simulink model "ECONANAL"  (Simulink 4.00)
settings: Solver=VariableStepDiscrete  SolverMode=SingleTasking  StartTime=0.0  StopTime=0  FixedStep=0  MaxStep=1  RelTol=1e-3  AbsTol=1e-6
settings Model: SaveTime=off  SaveOutput=off  LimitDataPoints=off  RTWTemplateMakefile=grt_unix.tmf  BlockReductionOpt=off

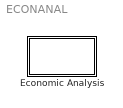
== system ECONANAL ==
  Economic Analysis : Subsystem
      settings: RTWFcnNameOpts=Auto  RTWFileNameOpts=Auto

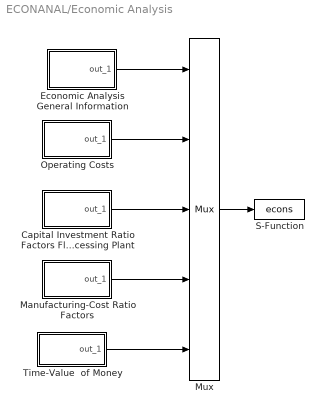
== system ECONANAL/Economic Analysis ==
  Capital Investment Ratio Factors Fluid Processing Plant : Subsystem
      settings: RTWFcnNameOpts=Auto  RTWFileNameOpts=Auto
  Economic Analysis General Information : Subsystem
      settings: RTWFcnNameOpts=Auto  RTWFileNameOpts=Auto
  Manufacturing-Cost Ratio Factors : Subsystem
      settings: RTWFcnNameOpts=Auto  RTWFileNameOpts=Auto
  Mux : Mux  Inputs=5
      settings: DisplayOption=none
  Operating Costs : Subsystem
      settings: RTWFcnNameOpts=Auto  RTWFileNameOpts=Auto
  S-Function : S-Function  FunctionName=econs  Parameters='ojstreams' 'ojunits'  PortCounts=[]  SFunctionModules=''
  Time-Value  of Money : Subsystem
      settings: RTWFcnNameOpts=Auto  RTWFileNameOpts=Auto
  wires:
  Economic Analysis General Information/1(out_1) -> Mux/1
  Mux/1 -> S-Function/1
  Time-Value  of Money/1(out_1) -> Mux/5
  Manufacturing-Cost Ratio Factors/1(out_1) -> Mux/4
  Capital Investment Ratio Factors Fluid Processing Plant/1(out_1) -> Mux/3
  Operating Costs/1(out_1) -> Mux/2

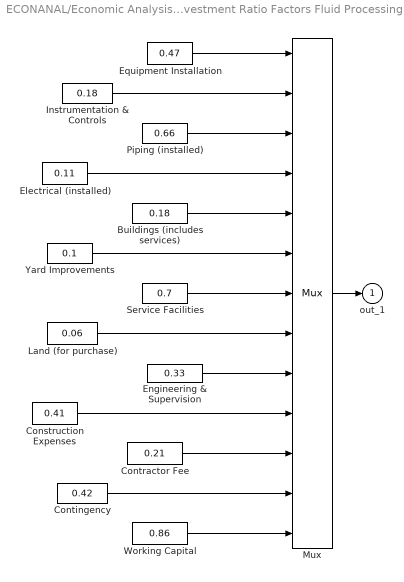
== system ECONANAL/Economic Analysis/Capital Investment Ratio Factors Fluid Processing Plant ==
  Buildings (includes services) : Constant  Value=0.18
  Construction Expenses : Constant  Value=0.41
  Contingency : Constant  Value=0.42
  Contractor Fee : Constant  Value=0.21
  Electrical (installed) : Constant  Value=0.11
  Engineering & Supervision : Constant  Value=0.33
  Equipment Installation : Constant  Value=0.47
  Instrumentation & Controls : Constant  Value=0.18
  Land (for purchase) : Constant  Value=0.06
  Mux : Mux  Inputs=13
      settings: DisplayOption=none
  Piping (installed) : Constant  Value=0.66
  Service Facilities : Constant  Value=0.7
  Working Capital : Constant  Value=0.86
  Yard Improvements : Constant  Value=0.1
  out_1 : Outport  Port=1  InitialOutput=0
  wires:
  Working Capital/1 -> Mux/13
  Contingency/1 -> Mux/12
  Contractor Fee/1 -> Mux/11
  Construction Expenses/1 -> Mux/10
  Engineering & Supervision/1 -> Mux/9
  Land (for purchase)/1 -> Mux/8
  Service Facilities/1 -> Mux/7
  Yard Improvements/1 -> Mux/6
  Buildings (includes services)/1 -> Mux/5
  Electrical (installed)/1 -> Mux/4
  Piping (installed)/1 -> Mux/3
  Instrumentation & Controls/1 -> Mux/2
  Equipment Installation/1 -> Mux/1
  Mux/1 -> out_1/1

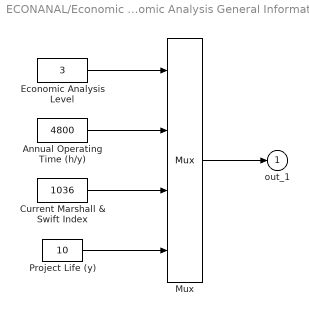
== system ECONANAL/Economic Analysis/Economic Analysis General Information ==
  Annual Operating Time (h/y) : Constant  Value=4800
  Current Marshall & Swift Index : Constant  Value=1036
  Economic Analysis Level : Constant  Value=3
  Mux : Mux  Inputs=4
      settings: DisplayOption=none
  Project Life (y) : Constant  Value=10
  out_1 : Outport  Port=1  InitialOutput=0
  wires:
  Mux/1 -> out_1/1
  Annual Operating Time (h/y)/1 -> Mux/2
  Current Marshall & Swift Index/1 -> Mux/3
  Economic Analysis Level/1 -> Mux/1
  Project Life (y)/1 -> Mux/4

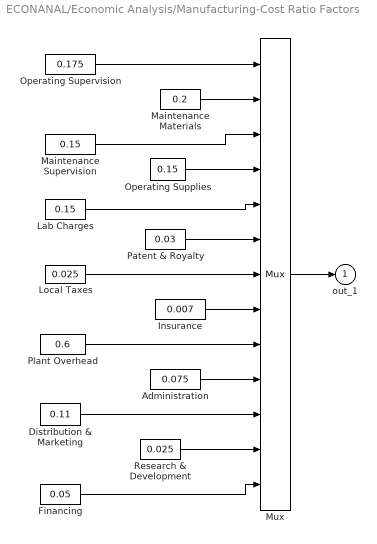
== system ECONANAL/Economic Analysis/Manufacturing-Cost Ratio Factors ==
  Administration : Constant  Value=0.075
  Distribution & Marketing : Constant  Value=0.11
  Financing : Constant  Value=0.05
  Insurance : Constant  Value=0.007
  Lab Charges : Constant  Value=0.15
  Local Taxes : Constant  Value=0.025
  Maintenance Materials : Constant  Value=0.2
  Maintenance Supervision : Constant  Value=0.15
  Mux : Mux  Inputs=13
      settings: DisplayOption=none
  Operating Supervision : Constant  Value=0.175
  Operating Supplies : Constant  Value=0.15
  Patent & Royalty : Constant  Value=0.03
  Plant Overhead : Constant  Value=0.6
  Research & Development : Constant  Value=0.025
  out_1 : Outport  Port=1  InitialOutput=0
  wires:
  Financing/1 -> Mux/13
  Research & Development/1 -> Mux/12
  Distribution & Marketing/1 -> Mux/11
  Administration/1 -> Mux/10
  Plant Overhead/1 -> Mux/9
  Insurance/1 -> Mux/8
  Local Taxes/1 -> Mux/7
  Patent & Royalty/1 -> Mux/6
  Lab Charges/1 -> Mux/5
  Operating Supplies/1 -> Mux/4
  Maintenance Supervision/1 -> Mux/3
  Maintenance Materials/1 -> Mux/2
  Operating Supervision/1 -> Mux/1
  Mux/1 -> out_1/1

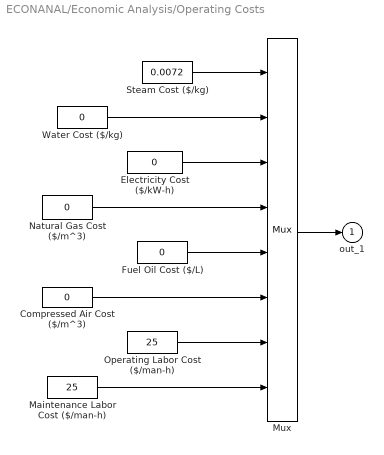
== system ECONANAL/Economic Analysis/Operating Costs ==
  Compressed Air Cost ($/m^3) : Constant  Value=0
  Electricity Cost ($/kW-h) : Constant  Value=0
  Fuel Oil Cost ($/L) : Constant  Value=0
  Maintenance Labor Cost ($/man-h) : Constant  Value=25
  Mux : Mux  Inputs=8
      settings: DisplayOption=none
  Natural Gas Cost ($/m^3) : Constant  Value=0
  Operating Labor Cost ($/man-h) : Constant  Value=25
  Steam Cost ($/kg) : Constant  Value=0.0072
  Water Cost ($/kg) : Constant  Value=0
  out_1 : Outport  Port=1  InitialOutput=0
  wires:
  Mux/1 -> out_1/1
  Steam Cost ($/kg)/1 -> Mux/1
  Water Cost ($/kg)/1 -> Mux/2
  Electricity Cost ($/kW-h)/1 -> Mux/3
  Natural Gas Cost ($/m^3)/1 -> Mux/4
  Fuel Oil Cost ($/L)/1 -> Mux/5
  Compressed Air Cost ($/m^3)/1 -> Mux/6
  Operating Labor Cost ($/man-h)/1 -> Mux/7
  Maintenance Labor Cost ($/man-h)/1 -> Mux/8

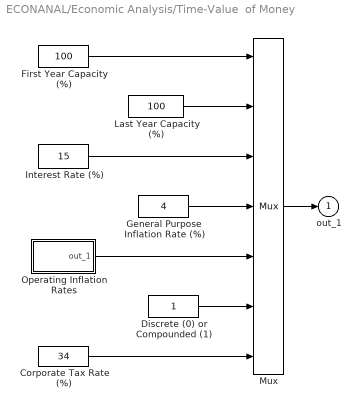
== system ECONANAL/Economic Analysis/Time-Value  of Money ==
  Corporate Tax Rate (%) : Constant  Value=34
  Discrete (0) or Compounded (1) : Constant  Value=1
  First Year Capacity (%) : Constant  Value=100
  General Purpose Inflation Rate (%) : Constant  Value=4
  Interest Rate (%) : Constant  Value=15
  Last Year Capacity (%) : Constant  Value=100
  Mux : Mux  Inputs=7
      settings: DisplayOption=none
  Operating Inflation Rates : Subsystem
      settings: RTWFcnNameOpts=Auto  RTWFileNameOpts=Auto
  out_1 : Outport  Port=1  InitialOutput=0
  wires:
  Mux/1 -> out_1/1
  First Year Capacity (%)/1 -> Mux/1
  Last Year Capacity (%)/1 -> Mux/2
  Interest Rate (%)/1 -> Mux/3
  General Purpose Inflation Rate (%)/1 -> Mux/4
  Operating Inflation Rates/1(out_1) -> Mux/5
  Discrete (0) or Compounded (1)/1 -> Mux/6
  Corporate Tax Rate (%)/1 -> Mux/7

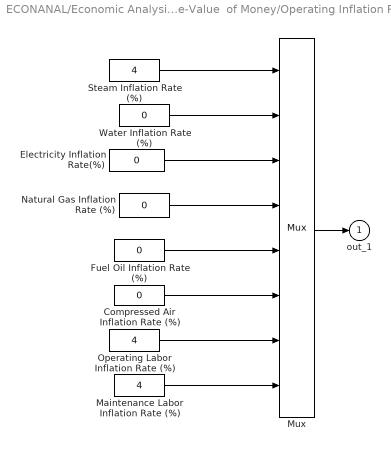
== system ECONANAL/Economic Analysis/Time-Value  of Money/Operating Inflation Rates ==
  Compressed Air Inflation Rate (%) : Constant  Value=0
  Electricity Inflation Rate(%) : Constant  Value=0
  Fuel Oil Inflation Rate (%) : Constant  Value=0
  Maintenance Labor Inflation Rate (%) : Constant  Value=4
  Mux : Mux  Inputs=8
      settings: DisplayOption=none
  Natural Gas Inflation Rate (%) : Constant  Value=0
  Operating Labor Inflation Rate (%) : Constant  Value=4
  Steam Inflation Rate (%) : Constant  Value=4
  Water Inflation Rate (%) : Constant  Value=0
  out_1 : Outport  Port=1  InitialOutput=0
  wires:
  Maintenance Labor Inflation Rate (%)/1 -> Mux/8
  Operating Labor Inflation Rate (%)/1 -> Mux/7
  Compressed Air Inflation Rate (%)/1 -> Mux/6
  Fuel Oil Inflation Rate (%)/1 -> Mux/5
  Natural Gas Inflation Rate (%)/1 -> Mux/4
  Electricity Inflation Rate(%)/1 -> Mux/3
  Water Inflation Rate (%)/1 -> Mux/2
  Steam Inflation Rate (%)/1 -> Mux/1
  Mux/1 -> out_1/1
